simulink model "angleSimulation"  (R2026a)
settings: Solver=VariableStepAuto
libraries: cstblocks_lti x3
settings Model: Creator=Maria  LastModifiedBy=Maria

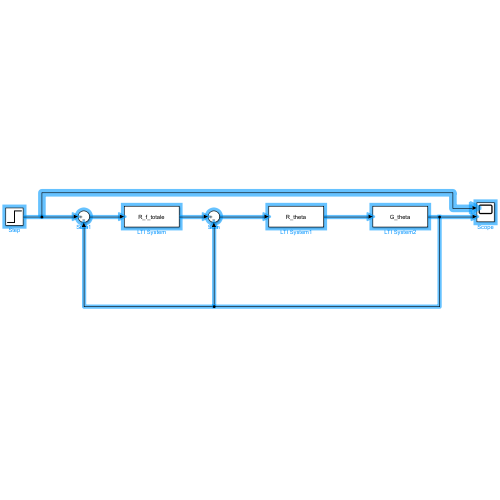
[thumbnail: Simulink's stored preview of the top-level diagram]
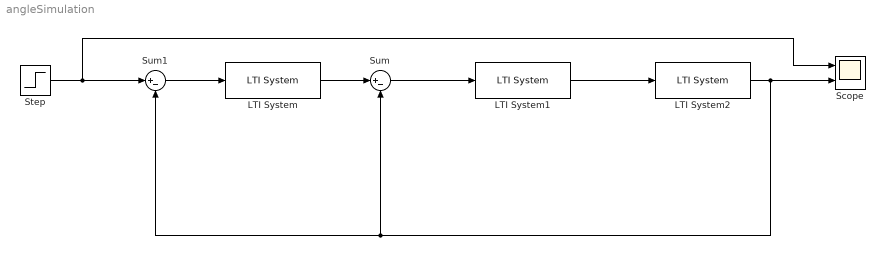
== system angleSimulation ==
  LTI System : cstblocks_lti/LTI System  sys=R_f_totale  IC=[]  PadeOrder=0
      settings: LibrarySourceBlock=cstblocks/LTI System
  LTI System1 : cstblocks_lti/LTI System  sys=R_theta  IC=[]  PadeOrder=0
      settings: LibrarySourceBlock=cstblocks/LTI System
  LTI System2 : cstblocks_lti/LTI System  sys=G_theta  IC=[]  PadeOrder=0
      settings: LibrarySourceBlock=cstblocks/LTI System
  Scope : Scope  NumInputPorts=2
      settings: ActiveDisplayYMinimum=-1  ActiveDisplayYMaximum=1
  Step : Step  FinalValue=0.1  SampleTime=0
  Sum : Sum  Inputs=|+-
  Sum1 : Sum  Inputs=|+-
  wires:
  LTI System/1 -> Sum/1
  Sum/1 -> LTI System1/1
  LTI System1/1 -> LTI System2/1
  Sum1/1 -> LTI System/1
  LTI System2/1 -> Sum1/2, Sum/2, Scope/2
  Step/1 -> Scope/1, Sum1/1
